simulink model "as2"  (R2023b)
settings: Solver=VariableStepAuto  StartTime=0.0  StopTime=10.0  RelTol=1e-3
undefined symbols (not defined in the file or in its folder): x
settings Model: Creator=mfb36  LastModifiedBy=mfb36

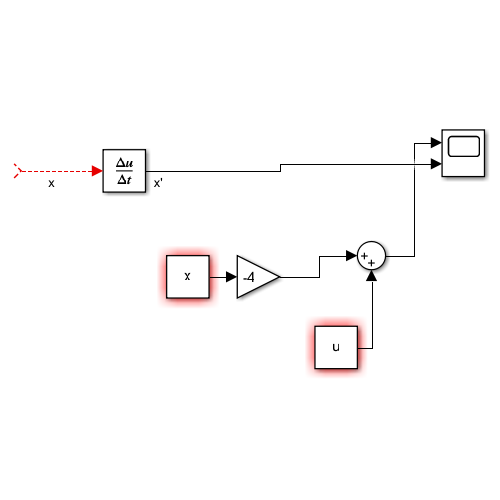
[thumbnail: Simulink's stored preview of the top-level diagram]
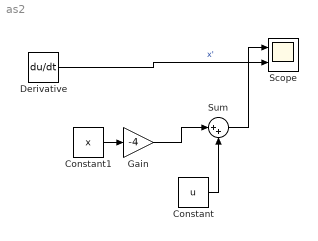
== system as2 ==
  Constant : Constant  Value=u
  Constant1 : Constant  Value=x
  Derivative : Derivative
  Gain : Gain  Gain=-4
  Scope : Scope  NumInputPorts=2
  Sum : Sum  Inputs=|++
  wires:
  ? -> Derivative/1  "x"
  Derivative/1 -> Scope/2  "x'"
  Constant1/1 -> Gain/1
  Constant/1 -> Sum/2
  Gain/1 -> Sum/1
  Sum/1 -> Scope/1
